simulink model "ctrl_ez"  (R2024b)
settings: configuration reference "CONFI" (kept outside this file)
InitFcn:
  | fidelity_pfc_vals;
  | wl=2*pi*50*150e-6;
  | 
  | gain_vac=1/(220*sqrt(2));
  | kpd = 5;
  | kpq = 5;
  | 
  | 
  | kid   =  1e2;
  | kiq   =  1e2;
  | 
  | kpvdc = .3;
  | kivdc =  .001;
values from neighbouring files (symbols this model uses):
  cos_th = cos(2*pi*50*t)    [fidelity_pfc_vals.m]
  sin_th = sin(2*pi*50*t)    [fidelity_pfc_vals.m]
  sin_th_vb = sin((2*pi*50*t)-(2*pi/3))    [fidelity_pfc_vals.m]
  sin_th_vc = sin((2*pi*50*t)+(2*pi/3))    [fidelity_pfc_vals.m]
  ts = 0.0001    [dic_pfc3ph.sldd]    (also in dictionary.sldd)
  tsw = 1/(fsw*1e3)    (= 1.53846153846e-05)    [fidelity_pfc_vals.m]
undefined symbols (not defined in the file or in its folder): DiscIntNeverNeededParam
libraries: mcbcontrolslib x18, simulink x5, dspswit3 x4, simulink_extras x2, slpidlib x2
(part 1 of 2)
settings Model: DataDictionary=dic_pfc3ph.sldd  Creator=Angel  LastModifiedBy=Angel
settings ConfigSetRef: SourceName=CONFI

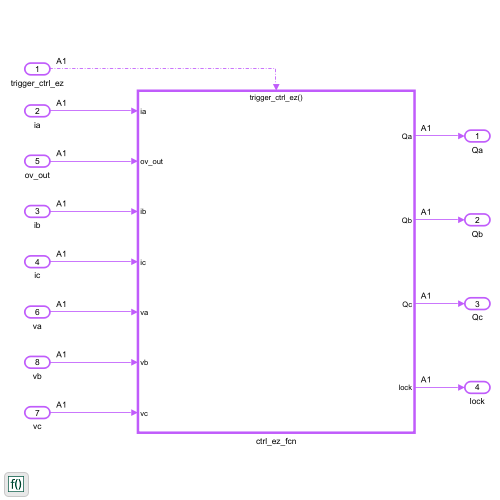
[thumbnail: Simulink's stored preview of the top-level diagram]
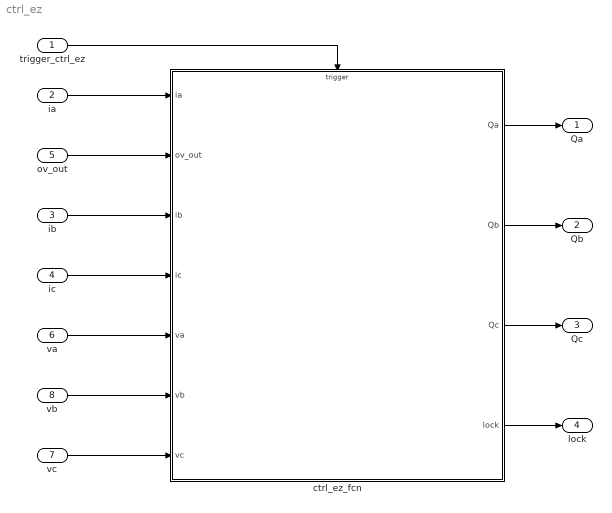
== system ctrl_ez ==
  trigger_ctrl_ez : Inport  OutputFunctionCall=on
  ia : Inport  Port=2
  ib : Inport  Port=3
  ic : Inport  Port=4
  ov_out : Inport  Port=5
  va : Inport  Port=6
  vc : Inport  Port=7
  vb : Inport  Port=8
  ctrl_ez_fcn : Subsystem
      settings: RTWSystemCode=Inline  RTWFcnNameOpts=Use subsystem name  RTWFileNameOpts=Use subsystem name  RTWMemSecFuncInitTerm=Default  RTWMemSecFuncExecute=Default
  Qa : Outport  PortDimensions=1
  Qb : Outport  Port=2
  Qc : Outport  Port=3
  lock : Outport  Port=4
  wires:
  ov_out/1 -> ctrl_ez_fcn/2(ov_out)
  trigger_ctrl_ez/1 -> ctrl_ez_fcn/Trigger
  va/1 -> ctrl_ez_fcn/5(va)
  ia/1 -> ctrl_ez_fcn/1(ia)
  vc/1 -> ctrl_ez_fcn/7(vc)
  ib/1 -> ctrl_ez_fcn/3(ib)
  vb/1 -> ctrl_ez_fcn/6(vb)
  ic/1 -> ctrl_ez_fcn/4(ic)
  ctrl_ez_fcn/1(Qa) -> Qa/1
  ctrl_ez_fcn/2(Qb) -> Qb/1
  ctrl_ez_fcn/3(Qc) -> Qc/1
  ctrl_ez_fcn/4(lock) -> lock/1

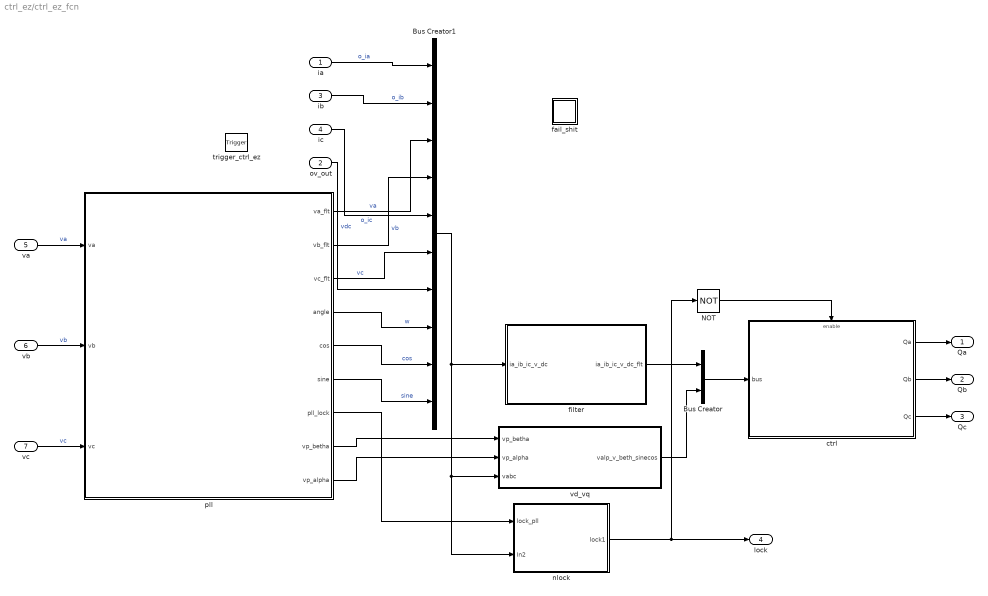
== system ctrl_ez/ctrl_ez_fcn ==
  ia : Inport  OutDataTypeStr=single
  ov_out : Inport  Port=2
  ib : Inport  Port=3  OutDataTypeStr=single
  ic : Inport  Port=4
  va : Inport  Port=5
  vb : Inport  Port=6
  vc : Inport  Port=7
  trigger_ctrl_ez : TriggerPort  TriggerType=function-call  VariantControl=(inherit)  PortDimensions=1
  Bus Creator : BusCreator  Inputs=2
  Bus Creator1 : BusCreator  Inputs=10
  NOT : Logic  Operator=NOT  IconShape=distinctive  AllPortsSameDT=off  OutDataTypeStr=boolean
  ctrl : Subsystem  TreatAsAtomicUnit=on
  fail_shit : Subsystem
  filter : Subsystem
  nlock : Subsystem
  pll : Subsystem
      settings: RTWSystemCode=Inline  RTWFcnNameOpts=Use subsystem name  RTWFileNameOpts=Use subsystem name  RTWMemSecFuncInitTerm=Default  RTWMemSecFuncExecute=Default
  vd_vq : Subsystem
  Qa : Outport
  Qb : Outport  Port=2
  Qc : Outport  Port=3
  lock : Outport  Port=4
  wires:
  ia/1 -> Bus Creator1/1  "o_ia"
  pll/3(vc_flt) -> Bus Creator1/6  "vc"
  pll/1(va_flt) -> Bus Creator1/3  "va"
  va/1 -> pll/1(va)  "va"
  ov_out/1 -> Bus Creator1/7  "vdc"
  vb/1 -> pll/2(vb)  "vb"
  ib/1 -> Bus Creator1/2  "o_ib"
  vc/1 -> pll/3(vc)  "vc"
  ic/1 -> Bus Creator1/5  "o_ic"
  ctrl/2(Qb) -> Qb/1
  pll/5(cos) -> Bus Creator1/9  "cos"
  pll/2(vb_flt) -> Bus Creator1/4  "vb"
  pll/6(sine) -> Bus Creator1/10  "sine"
  pll/4(angle) -> Bus Creator1/8  "w"
  pll/7(pll_lock) -> nlock/1(lock_pll)
  Bus Creator1/1 -> nlock/2(In2), vd_vq/3(vabc), filter/1(ia_ib_ic_v_dc)
  nlock/1(lock1) -> NOT/1, lock/1
  filter/1(ia_ib_ic_v_dc_flt) -> Bus Creator/1
  vd_vq/1(valp_v_beth_sinecos) -> Bus Creator/2
  NOT/1 -> ctrl/Enable
  Bus Creator/1 -> ctrl/1(bus)
  ctrl/1(Qa) -> Qa/1
  ctrl/3(Qc) -> Qc/1
  pll/8(vp_betha) -> vd_vq/1(vp_betha)
  pll/9(vp_alpha) -> vd_vq/2(vp_alpha)

== system ctrl_ez/ctrl_ez_fcn/ctrl ==
  bus : Inport
  Enable : EnablePort
  id_iq : Subsystem
  pi_ctrl : Subsystem
  svm : Subsystem
  Qa : Outport
  Qb : Outport  Port=2
  Qc : Outport  Port=3
  wires:
  id_iq/1(id) -> pi_ctrl/1(id)
  bus/1 -> svm/3(bus), pi_ctrl/3(bus), id_iq/1(In3)
  id_iq/2(iq) -> pi_ctrl/2(iq)
  svm/1(Qa) -> Qa/1
  svm/2(Qb) -> Qb/1
  svm/3(Qc) -> Qc/1
  pi_ctrl/1(d) -> svm/1(d)
  pi_ctrl/2(q) -> svm/2(q)

== system ctrl_ez/ctrl_ez_fcn/fail_shit ==
  pi+svpwm : Subsystem  Commented=on
  pi+svpwm1 : Subsystem  Commented=on

== system ctrl_ez/ctrl_ez_fcn/filter ==
  ia_ib_ic_v_dc : Inport
  Bus Creator : BusCreator  Inputs=3
  Bus Selector : BusSelector  OutputSignals=o_ia,o_ib,o_ic  OutputAsBus=on
  Data Store Memory : DataStoreMemory  DataStoreName=filter_IA  WriteAfterWriteMsg=warning  ShowAdditionalParam=off  StateMustResolveToSignalObject=on
  Data Store Memory1 : DataStoreMemory  DataStoreName=filter_IB  WriteAfterWriteMsg=warning  ShowAdditionalParam=off  StateMustResolveToSignalObject=on
  Data Store Memory2 : DataStoreMemory  DataStoreName=filter_IC  WriteAfterWriteMsg=warning  ShowAdditionalParam=off  StateMustResolveToSignalObject=on
  Data Store Write : DataStoreWrite  DataStoreName=filter_IA  IndexOptions=Index vector (dialog)  Indices=1  OutputSizes=1
  Data Store Write1 : DataStoreWrite  DataStoreName=filter_IB  IndexOptions=Index vector (dialog)  Indices=1  OutputSizes=1
  Data Store Write2 : DataStoreWrite  DataStoreName=filter_IC  IndexOptions=Index vector (dialog)  Indices=1  OutputSizes=1
  Demux : Demux  Outputs=3
  IIR Filter : mcbcontrolslib/IIR Filter  Commented=through  VariantControl=Low Pass Filter  VariantSelect=Low-pass  FilterConstantInputType=Specify via dialog  Filter_constant=.1  advancedSettings=on  Ts=1/8e3  cutOff_freq=141.4711
  ia_ib_ic_v_dc_flt : Outport
  wires:
  ia_ib_ic_v_dc/1 -> Bus Selector/1
  IIR Filter/1 -> Demux/1
  Bus Selector/1 -> IIR Filter/1
  Demux/1 -> Data Store Write/1, Bus Creator/1  "flt_ia"
  Demux/2 -> Data Store Write1/1, Bus Creator/2  "flt_ib"
  Demux/3 -> Data Store Write2/1, Bus Creator/3  "flt_ic"
  Bus Creator/1 -> ia_ib_ic_v_dc_flt/1

== system ctrl_ez/ctrl_ez_fcn/nlock ==
  lock_pll : Inport
  In2 : Inport  Port=2
  AND : Logic  IconShape=distinctive  AllPortsSameDT=off  OutDataTypeStr=boolean
  Bus Selector : BusSelector  OutputSignals=w
  Constant : Constant  Value=0  OutDataTypeStr=boolean  SampleTime=-1
  Equal : RelationalOperator  Operator=>  OutDataTypeStr=boolean  RndMeth=Simplest  InputSameDT=off
  Memory : Memory  InitialCondition=1  InheritSampleTime=on
  Pi1 : Constant  Value=0  OutDataTypeStr=single  SampleTime=-1
  Switch : Switch  Criteria=u2 > Threshold  SaturateOnIntegerOverflow=off  InputSameDT=off
  lock1 : Outport
  wires:
  Switch/1 -> lock1/1, Memory/1
  Constant/1 -> Switch/1
  Memory/1 -> Switch/3
  In2/1 -> Bus Selector/1
  Bus Selector/1 -> Equal/1  "<w>"
  Equal/1 -> AND/1
  Pi1/1 -> Equal/2
  lock_pll/1 -> AND/2
  AND/1 -> Switch/2

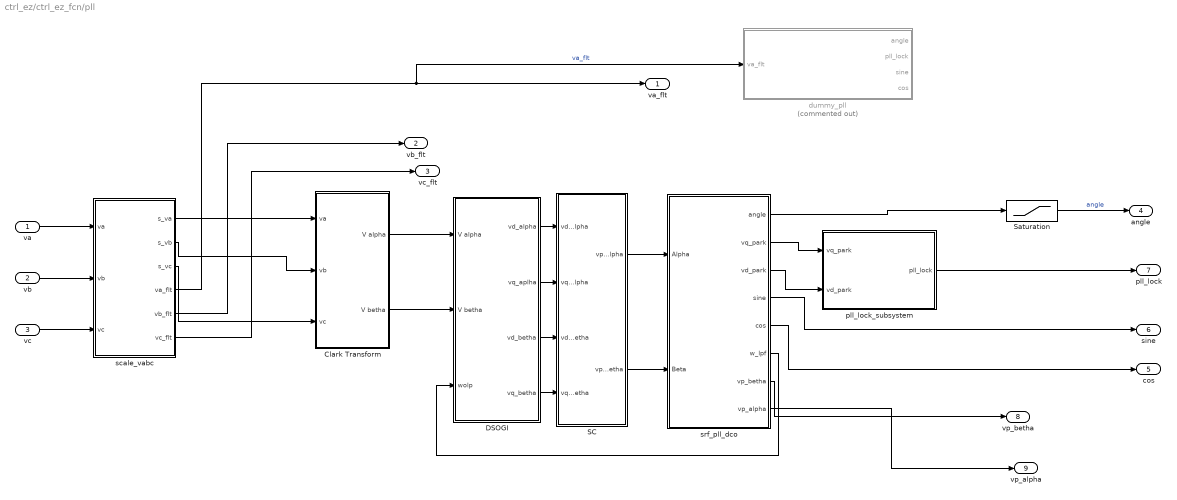
== system ctrl_ez/ctrl_ez_fcn/pll ==
  va : Inport  OutDataTypeStr=single
  vb : Inport  Port=2  OutDataTypeStr=single
  vc : Inport  Port=3  OutDataTypeStr=single
  Clark Transform : Subsystem  SystemSampleTime=ts
  DSOGI : Subsystem  SystemSampleTime=ts
  SC : Subsystem  SystemSampleTime=ts
  Saturation : Saturate  UpperLimit=2*pi  LowerLimit=0
  dummy_pll : Subsystem  Commented=on
  pll_lock_subsystem : Subsystem
  scale_vabc : Subsystem
  srf_pll_dco : Subsystem
  va_flt : Outport
  vb_flt : Outport  Port=2
  vc_flt : Outport  Port=3
  angle : Outport  Port=4
  cos : Outport  Port=5
  sine : Outport  Port=6
  pll_lock : Outport  Port=7
  vp_betha : Outport  Port=8
  vp_alpha : Outport  Port=9
  wires:
  vb/1 -> scale_vabc/2(vb)
  scale_vabc/3(s_vc) -> Clark Transform/3(vc)
  scale_vabc/2(s_vb) -> Clark Transform/2(vb)
  srf_pll_dco/5(cos) -> cos/1
  pll_lock_subsystem/1(pll_lock) -> pll_lock/1
  srf_pll_dco/2(vq_park) -> pll_lock_subsystem/1(vq_park)
  SC/2(vp_betha) -> srf_pll_dco/2(Beta)
  SC/1(vp_alpha) -> srf_pll_dco/1(Alpha)
  DSOGI/2(vq_aplha) -> SC/2(vq_sogi_alpha)
  DSOGI/1(vd_alpha) -> SC/1(vd_sogi_alpha)
  srf_pll_dco/3(vd_park) -> pll_lock_subsystem/2(vd_park)
  srf_pll_dco/6(w_lpf) -> DSOGI/3(wolp)
  va/1 -> scale_vabc/1(va)
  Clark Transform/2(V betha) -> DSOGI/2(V betha)
  scale_vabc/1(s_va) -> Clark Transform/1(va)
  srf_pll_dco/4(sine) -> sine/1
  srf_pll_dco/1(angle) -> Saturation/1
  DSOGI/3(vd_betha) -> SC/3(vd_sogi_betha)
  Clark Transform/1(V alpha) -> DSOGI/1(V alpha)
  DSOGI/4(vq_betha) -> SC/4(vq_sogi_betha)
  vc/1 -> scale_vabc/3(vc)
  scale_vabc/4(va_flt) -> dummy_pll/1(va_flt), va_flt/1  "va_flt"
  scale_vabc/5(vb_flt) -> vb_flt/1
  scale_vabc/6(vc_flt) -> vc_flt/1
  Saturation/1 -> angle/1  "angle"
  srf_pll_dco/7(vp_betha) -> vp_betha/1
  srf_pll_dco/8(vp_alpha) -> vp_alpha/1

== system ctrl_ez/ctrl_ez_fcn/vd_vq ==
  vp_betha : Inport
  vp_alpha : Inport  Port=2
  vabc : Inport  Port=3
  Bus Creator : BusCreator  Inputs=3
  Bus Creator1 : BusCreator  Inputs=2
  Bus Selector : BusSelector  OutputSignals=w,vc,vb,va,cos,sine
  Clarke Transform : mcbcontrolslib/Clarke Transform  Commented=on  VariantControl=Variant2  PhaseInput=Three inputs  EnPowerInv=on
      settings: LibrarySourceBlock=mcbhdllib/Controls/Math Transforms/Clarke Transform
  Demux : Demux  Commented=on  Outputs=3
  Mux : Mux  Commented=on  Inputs=3
  Park Transform : mcbcontrolslib/Park Transform  Commented=on  PhaseInput=Two inputs  AxisAlignment=Q-axis  ThetaInput=Sine and Cosine electrical position  AngleInput=Radians  N_points=1024
  Terminator : Terminator  Commented=on
  park_tf : MATLAB Function  Commented=on  TreatAsAtomicUnit=on  VariantControl=false()
  valp_v_beth_sinecos : Outport
  wires:
  vabc/1 -> Bus Creator1/2, Bus Selector/1
  vp_alpha/1 -> Bus Creator/1  "vd_"
  vp_betha/1 -> Bus Creator/2  "vq_"
  Bus Selector/1 -> Bus Creator/3  "<w>"
  Bus Creator/1 -> Bus Creator1/1
  Bus Creator1/1 -> valp_v_beth_sinecos/1
  Bus Selector/5 -> Park Transform/4, park_tf/4(cos_th_k_1)  "<cos>"
  Bus Selector/6 -> Park Transform/3, park_tf/3(sin_th_k_1)  "<sine>"
  Mux/1 -> Clarke Transform/1
  Demux/3 -> Terminator/1
  Clarke Transform/1 -> Demux/1
  Demux/1 -> park_tf/1(vp_alpha)
  Demux/2 -> park_tf/2(vp_betha)
  Bus Selector/2 -> Mux/3  "<vc>"
  Bus Selector/3 -> Mux/2  "<vb>"
  Bus Selector/4 -> Mux/1  "<va>"

== system ctrl_ez/ctrl_ez_fcn/ctrl/id_iq ==
  In3 : Inport
  Bus Selector1 : BusSelector  OutputSignals=signal1.flt_ia,signal1.flt_ib,signal1.flt_ic,signal2.signal2.cos,signal2.signal2.sine
  Clarke Transform : mcbcontrolslib/Clarke Transform  VariantControl=Variant2  PhaseInput=Three inputs  EnPowerInv=on
      settings: LibrarySourceBlock=mcbhdllib/Controls/Math Transforms/Clarke Transform
  Demux1 : Demux  Outputs=3
  Mux : Mux  Inputs=3
  Terminator1 : Terminator
  park_tf : MATLAB Function  TreatAsAtomicUnit=on  VariantControl=false()
  id : Outport
  iq : Outport  Port=2
  wires:
  In3/1 -> Bus Selector1/1
  Demux1/2 -> park_tf/2(vp_betha)  "iq"
  Clarke Transform/1 -> Demux1/1
  Bus Selector1/1 -> Mux/1  "<flt_ia>"
  Mux/1 -> Clarke Transform/1
  Bus Selector1/2 -> Mux/2  "<flt_ib>"
  Bus Selector1/3 -> Mux/3  "<flt_ic>"
  Demux1/1 -> park_tf/1(vp_alpha)  "id"
  Demux1/3 -> Terminator1/1
  park_tf/1(vd_park) -> id/1  "id"
  park_tf/2(vq_park) -> iq/1  "iq"
  Bus Selector1/4 -> park_tf/4(cos_th_k_1)  "<cos>"
  Bus Selector1/5 -> park_tf/3(sin_th_k_1)  "<sine>"

== system ctrl_ez/ctrl_ez_fcn/ctrl/pi_ctrl ==
  id : Inport
  iq : Inport  Port=2
  bus : Inport  Port=3
  Bus Selector2 : BusSelector  OutputSignals=signal2.signal1.vd_,signal2.signal1.vq_,signal2.signal2.vdc
  Constant : Constant  Value=650  OutDataTypeStr=single  SampleTime=-1
  Constant1 : Constant  Value=0  OutDataTypeStr=single  SampleTime=-1
  Gain : Gain  Gain=wl
  Gain1 : Gain  Gain=wl
  Sum1 : Sum  Inputs=|+-
  Sum2 : Sum  Inputs=|+-
  Sum3 : Sum  Inputs=++-
  Sum4 : Sum  Inputs=-|+||
  Sum5 : Sum  Inputs=+--
  id_ctrl : Subsystem  SystemSampleTime=tsw
  iq_ctrl : Subsystem  SystemSampleTime=tsw
  speed_ctrl : Subsystem  SystemSampleTime=tsw
  d : Outport
  q : Outport  Port=2
  wires:
  Constant/1 -> Sum1/1
  Sum1/1 -> speed_ctrl/1(i_error)  "vdc_error"
  iq/1 -> Sum4/1, Gain/1  "iq"
  speed_ctrl/1(I_D_CTRL_VDC) -> Sum2/1  "id_ctrl"
  Constant1/1 -> Sum4/2  "vq_ctrl"
  id/1 -> Sum2/2, Gain1/1  "id"
  Sum4/1 -> iq_ctrl/1(i_error)  "iq_error"
  Sum2/1 -> id_ctrl/1(i_error)  "id_error"
  Gain1/1 -> Sum5/2  "idwl"
  iq_ctrl/1(v_ind) -> Sum5/3  "vq_ctrl"
  Gain/1 -> Sum3/2  "iqwl"
  id_ctrl/1(v_ind) -> Sum3/3  "vd_ctrl"
  Sum5/1 -> q/1  "vq_ctrl"
  Sum3/1 -> d/1  "vd_ctrl"
  bus/1 -> Bus Selector2/1
  Bus Selector2/3 -> Sum1/2  "<vdc>"
  Bus Selector2/1 -> Sum3/1  "<vd_>"
  Bus Selector2/2 -> Sum5/1  "<vq_>"

== system ctrl_ez/ctrl_ez_fcn/ctrl/svm ==
  d : Inport
  q : Inport  Port=2
  bus : Inport  Port=3
  Bus Selector : BusSelector  OutputSignals=signal2.signal2.cos,signal2.signal2.sine,signal2.signal2.w,signal2.signal2.vdc
  mine_invpark_tf : MATLAB Function  TreatAsAtomicUnit=on  VariantControl=false()
  pi+svpwm1 : Subsystem  Commented=on
  relat_time : Subsystem
  section_cal : Subsystem
  threshold : Subsystem
  Qa : Outport
  Qb : Outport  Port=2
  Qc : Outport  Port=3
  wires:
  mine_invpark_tf/1(vp_alpha) -> section_cal/2(v_alp)  "vind_alp"
  mine_invpark_tf/2(vp_betha) -> section_cal/3(v_bet)  "vind_bet"
  section_cal/1(alpha) -> relat_time/2(alpha)
  threshold/3(qc) -> Qc/1
  section_cal/2(oddsect) -> relat_time/3(odd_section)
  threshold/2(qb) -> Qb/1
  section_cal/3(vs_mag) -> relat_time/4(vs_mag)
  relat_time/1(ta_tb_t0) -> threshold/1(ta_tb_t0)
  section_cal/4(SA SB SC) -> threshold/2(SA SB SC)
  threshold/1(qa) -> Qa/1
  bus/1 -> Bus Selector/1
  d/1 -> mine_invpark_tf/1(vd_park)
  q/1 -> mine_invpark_tf/2(vq_park)
  Bus Selector/1 -> mine_invpark_tf/4(cos_th_k_1)  "<cos>"
  Bus Selector/2 -> mine_invpark_tf/3(sin_th_k_1)  "<sine>"
  Bus Selector/3 -> section_cal/1(<w>)  "<w>"
  Bus Selector/4 -> relat_time/1(vdc)  "<vdc>"

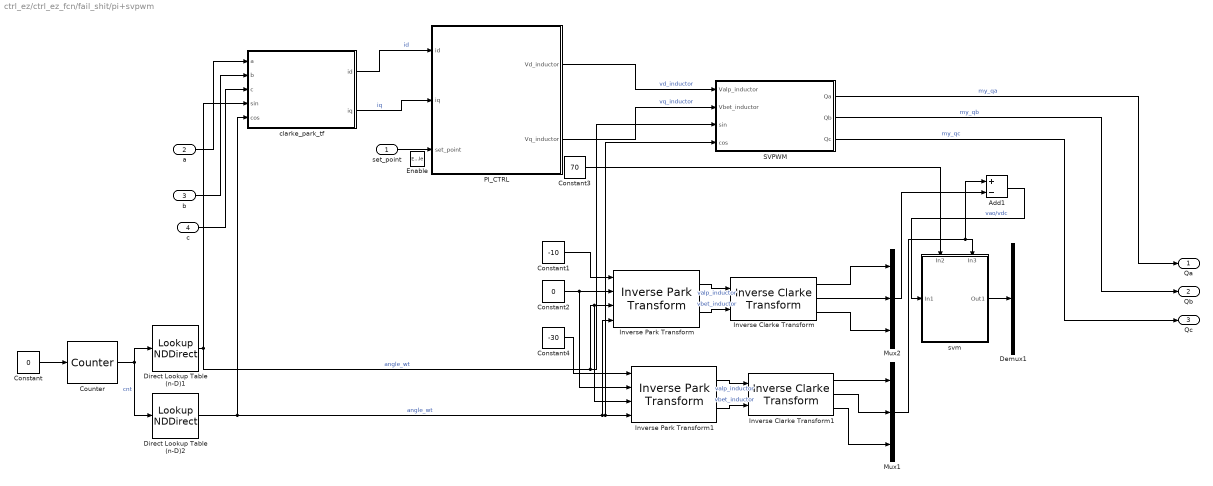
== system ctrl_ez/ctrl_ez_fcn/fail_shit/pi+svpwm ==
  set_point : Inport
  a : Inport  Port=2
  b : Inport  Port=3
  c : Inport  Port=4
  Enable : EnablePort
  Add1 : Sum  Inputs=+-
  Constant : Constant  Value=0  SampleTime=-1
  Constant1 : Constant  Value=-10
  Constant2 : Constant  Value=0
  Constant3 : Constant  Value=70
  Constant4 : Constant  Value=-30
  Counter : dspswit3/Counter  Direction=Up  CountEvent=Free running  CounterSize=User defined  MaxCount=(.01/tsw)+1  InitialCount=0  Output=Count  HitValue=32  ResetInput=on  SamplesPerFrame=1  Ts=-1  CntDtype=uint32  HitDtype=Logical
  Demux1 : Demux  Outputs=3
  Direct Lookup Table (n-D)1 : LookupNDDirect  NumberOfTableDimensions=1  Table=single(sin_th);  RemoveProtectionInput=on  TableDataTypeStr=single
  Direct Lookup Table (n-D)2 : LookupNDDirect  NumberOfTableDimensions=1  Table=single(cos_th);  RemoveProtectionInput=on  TableDataTypeStr=single
  Inverse Clarke Transform : mcbcontrolslib/Inverse Clarke Transform  PhaseInput=Two inputs  EnPowerInv=off
      settings: LibrarySourceBlock=mcbhdllib/Controls/Math Transforms/Inverse Clarke Transform
  Inverse Clarke Transform1 : mcbcontrolslib/Inverse Clarke Transform  PhaseInput=Two inputs  EnPowerInv=off
      settings: LibrarySourceBlock=mcbhdllib/Controls/Math Transforms/Inverse Clarke Transform
  Inverse Park Transform : mcbcontrolslib/Inverse Park Transform  PhaseInput=Two inputs  AxisAlignment=D-axis  ThetaInput=Sine and Cosine electrical position  AngleInput=Per-unit  N_points=1024
      settings: LibrarySourceBlock=mcbhdllib/Controls/Math Transforms/Inverse Park Transform
  Inverse Park Transform1 : mcbcontrolslib/Inverse Park Transform  PhaseInput=Two inputs  AxisAlignment=D-axis  ThetaInput=Sine and Cosine electrical position  AngleInput=Per-unit  N_points=1024
      settings: LibrarySourceBlock=mcbhdllib/Controls/Math Transforms/Inverse Park Transform
  Mux1 : Mux  Inputs=3
  Mux2 : Mux  Inputs=3
  PI_CTRL : Subsystem  SystemSampleTime=tsw
  SVPWM : Subsystem  SystemSampleTime=tsw
  clarke_park_tf : Subsystem
  svm : Subsystem
      settings: PortSchema="{\"entries\":[{\"content\":{\"sides\":[{\"content\":{\"connectorIds\":[\"In1\"]},\"type\":\"ConnectorPlacement.EquallySpacedRectSide\",\"uuid\":\"3e008ee5-59f8-4da6-a2e7-d375939bf865\"},{\"content\":{\"connectorIds\":[\"Out1\"],\"side\":\"RIGHT\"},\"type\":\"ConnectorPlacement.EquallySpacedRectSide\",\"uuid\":\"8b37db03-1d3b-40e7-b6c7-a20c319c3381\"},{\"content\":{\"connectorIds\":[\"In2\",\"In3\"],\"side\":\"TOP\"},\"type\":\"ConnectorPlacement.EquallySpacedRectSide\",\"uuid\":\"db383d90-c1d4-4862-ad96-70764e497fba\"}]},\"type\":\"ConnectorPlacement.EquallySpacedConnector\",\"uuid\":\"69b3b40e-ea56-4f3d-9cab-f35d699fcec1\"}],\"packageUris\":[\"http://schema.mathworks.com/mf0/Connector/R2020b\"],\"version\":\"1.0\"}"
  Qa : Outport
  Qb : Outport  Port=2
  Qc : Outport  Port=3
  wires:
  b/1 -> clarke_park_tf/2(b)
  c/1 -> clarke_park_tf/3(c)
  Constant/1 -> Counter/1
  Counter/1 -> Direct Lookup Table (n-D)2/1, Direct Lookup Table (n-D)1/1  "cnt"
  set_point/1 -> PI_CTRL/3(set_point)
  a/1 -> clarke_park_tf/1(a)
  clarke_park_tf/1(id) -> PI_CTRL/1(id)  "id"
  Direct Lookup Table (n-D)2/1 -> clarke_park_tf/5(cos), SVPWM/4(cos), Inverse Park Transform1/4, Inverse Park Transform/4  "angle_wt"
  Direct Lookup Table (n-D)1/1 -> SVPWM/3(sin), Inverse Park Transform1/3, Inverse Park Transform/3, clarke_park_tf/4(sin)  "angle_wt"
  clarke_park_tf/2(iq) -> PI_CTRL/2(iq)  "iq"
  Constant1/1 -> Inverse Park Transform/1
  Constant2/1 -> Inverse Park Transform1/2, Inverse Park Transform/2
  Constant3/1 -> svm/2(In2)
  Add1/1 -> svm/1(In1)  "vao/vdc"
  Mux2/1 -> Add1/2
  svm/1(Out1) -> Demux1/1
  Inverse Park Transform/2 -> Inverse Clarke Transform/2  "vbet_inductor"
  Inverse Park Transform/1 -> Inverse Clarke Transform/1  "valp_inductor"
  Inverse Clarke Transform/2 -> Mux2/2
  Inverse Clarke Transform/3 -> Mux2/3
  Inverse Clarke Transform/1 -> Mux2/1
  Inverse Park Transform1/1 -> Inverse Clarke Transform1/1  "valp_inductor"
  Inverse Park Transform1/2 -> Inverse Clarke Transform1/2  "vbet_inductor"
  Inverse Clarke Transform1/1 -> Mux1/1
  Inverse Clarke Transform1/2 -> Mux1/2
  Inverse Clarke Transform1/3 -> Mux1/3
  Mux1/1 -> Add1/1, svm/3(In3)
  Constant4/1 -> Inverse Park Transform1/1
  PI_CTRL/1(Vd_inductor) -> SVPWM/1(Valp_inductor)  "vd_inductor"
  PI_CTRL/2(Vq_inductor) -> SVPWM/2(Vbet_inductor)  "vq_inductor"
  SVPWM/1(Qa) -> Qa/1  "my_qa"
  SVPWM/2(Qb) -> Qb/1  "my_qb"
  SVPWM/3(Qc) -> Qc/1  "my_qc"

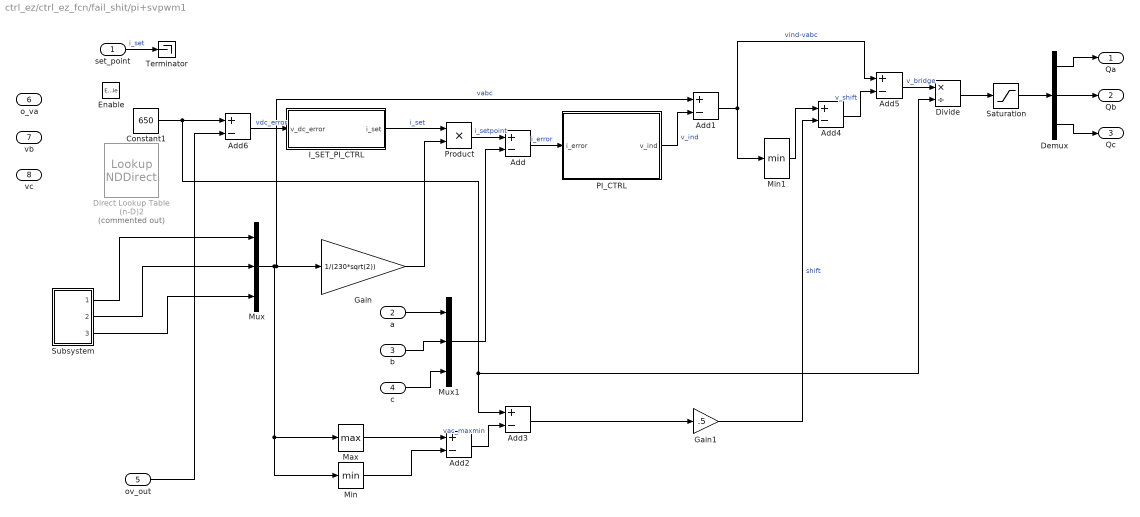
== system ctrl_ez/ctrl_ez_fcn/fail_shit/pi+svpwm1 ==
  set_point : Inport
  a : Inport  Port=2
  b : Inport  Port=3
  c : Inport  Port=4
  ov_out : Inport  Port=5
  o_va : Inport  Port=6
  vb : Inport  Port=7
  vc : Inport  Port=8
  Enable : EnablePort
  Add{,1..6} (7 alike) : Sum  Inputs=+-
  Constant1 : Constant  Value=650  VectorParams1D=off  OutDataTypeStr=single  SampleTime=-1
  Demux : Demux  Outputs=3
  Direct Lookup Table (n-D)2 : LookupNDDirect  Commented=on  NumberOfTableDimensions=1  Table=single(cos_th);  RemoveProtectionInput=on  TableDataTypeStr=single
  Divide : Product  Inputs=*/
  Gain : Gain  Gain=1/(230*sqrt(2))
  Gain1 : Gain  Gain=.5
  I_SET_PI_CTRL : Subsystem  SystemSampleTime=tsw
  Max : MinMax  Function=max
  Min : MinMax
  Min1 : MinMax
  Mux : Mux  Inputs=3
  Mux1 : Mux  Inputs=3
  PI_CTRL : Subsystem  SystemSampleTime=tsw
  Product : Product
  Saturation : Saturate  UpperLimit=.97  LowerLimit=.03
  Subsystem : Subsystem
  Terminator : Terminator
  Qa : Outport
  Qb : Outport  Port=2
  Qc : Outport  Port=3
  wires:
  Constant1/1 -> Add3/1, Divide/2, Add6/1
  ov_out/1 -> Add6/2
  Gain/1 -> Product/2
  Add6/1 -> I_SET_PI_CTRL/1(v_dc_error)  "vdc_error"
  b/1 -> Mux1/2
  Mux/1 -> Max/1, Min/1, Add1/1, Gain/1  "vabc"
  set_point/1 -> Terminator/1  "i_set"
  a/1 -> Mux1/1
  c/1 -> Mux1/3
  Max/1 -> Add2/1
  Min/1 -> Add2/2
  Product/1 -> Add/1  "i_setpoint"
  Mux1/1 -> Add/2
  Add2/1 -> Add3/2  "vac_maxmin"
  Add/1 -> PI_CTRL/1(i_error)  "i_error"
  Add3/1 -> Gain1/1
  PI_CTRL/1(v_ind) -> Add1/2  "v_ind"
  Add1/1 -> Add5/1, Min1/1  "vind-vabc"
  Gain1/1 -> Add4/2  "shift"
  Min1/1 -> Add4/1
  Add4/1 -> Add5/2  "v_shift"
  Add5/1 -> Divide/1  "v_bridge"
  Divide/1 -> Saturation/1
  Demux/2 -> Qb/1
  Demux/1 -> Qa/1
  Saturation/1 -> Demux/1
  Demux/3 -> Qc/1
  I_SET_PI_CTRL/1(i_set) -> Product/1  "i_set"
  Subsystem/1(angle_wt) -> Mux/1
  Subsystem/2(angle_wt1) -> Mux/2
  Subsystem/3(angle_wt2) -> Mux/3

== system ctrl_ez/ctrl_ez_fcn/pll/Clark Transform ==
  va : Inport  OutDataTypeStr=single
  vb : Inport  Port=2  OutDataTypeStr=single
  vc : Inport  Port=3  OutDataTypeStr=single
  Clarke Transform : mcbcontrolslib/Clarke Transform  VariantControl=Variant2  PhaseInput=Three inputs  EnPowerInv=on
      settings: LibrarySourceBlock=mcbhdllib/Controls/Math Transforms/Clarke Transform
  Demux : Demux  Outputs=3
  Mux : Mux  Inputs=3
  Terminator : Terminator
  V alpha : Outport
  V betha : Outport  Port=2
  wires:
  vb/1 -> Mux/2
  va/1 -> Mux/1
  Demux/3 -> Terminator/1
  Demux/2 -> V betha/1  "V betha_pll"
  Demux/1 -> V alpha/1  "V alpha_pll"
  vc/1 -> Mux/3
  Mux/1 -> Clarke Transform/1
  Clarke Transform/1 -> Demux/1

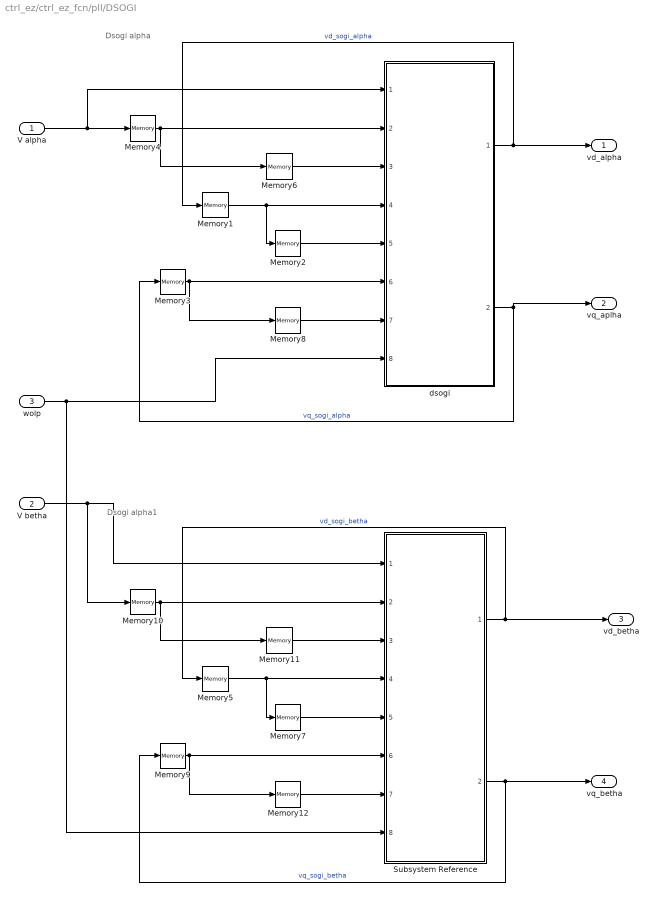
== system ctrl_ez/ctrl_ez_fcn/pll/DSOGI ==
  note: Dsogi alpha1
  note: Dsogi alpha
  V alpha : Inport  OutDataTypeStr=single
  V betha : Inport  Port=2  OutDataTypeStr=single
  wolp : Inport  Port=3  OutDataTypeStr=single
  Memory{1..12} (12 alike) : Memory  InheritSampleTime=on
  Subsystem Reference : Subsystem  ReferencedSubsystem=dsogi
  dsogi : Subsystem  ReferencedSubsystem=dsogi
  vd_alpha : Outport
  vq_aplha : Outport  Port=2
  vd_betha : Outport  Port=3
  vq_betha : Outport  Port=4
  wires:
  dsogi/2 -> vq_aplha/1, Memory3/1  "vq_sogi_alpha"
  dsogi/1 -> vd_alpha/1, Memory1/1  "vd_sogi_alpha"
  Memory8/1 -> dsogi/7
  Memory2/1 -> dsogi/5
  Memory6/1 -> dsogi/3
  Memory3/1 -> dsogi/6, Memory8/1
  Memory1/1 -> dsogi/4, Memory2/1
  Memory4/1 -> dsogi/2, Memory6/1
  V alpha/1 -> dsogi/1, Memory4/1
  Subsystem Reference/2 -> vq_betha/1, Memory9/1  "vq_sogi_betha"
  Subsystem Reference/1 -> vd_betha/1, Memory5/1  "vd_sogi_betha"
  wolp/1 -> Subsystem Reference/8, dsogi/8
  Memory12/1 -> Subsystem Reference/7
  Memory7/1 -> Subsystem Reference/5
  Memory11/1 -> Subsystem Reference/3
  V betha/1 -> Subsystem Reference/1, Memory10/1
  Memory10/1 -> Subsystem Reference/2, Memory11/1
  Memory5/1 -> Subsystem Reference/4, Memory7/1
  Memory9/1 -> Subsystem Reference/6, Memory12/1

== system ctrl_ez/ctrl_ez_fcn/pll/SC ==
  note: c=0.5*(a+b);
  note: c=0.5*(a-b);
  note: NSC
  vd_sogi_alpha : Inport  OutDataTypeStr=single
  vq_sogi_alpha : Inport  Port=2  OutDataTypeStr=single
  vd_sogi_betha : Inport  Port=3  OutDataTypeStr=single
  vq_sogi_betha : Inport  Port=4  OutDataTypeStr=single
  Add : Sum  Inputs=+-
  Add1 : Sum
  Gain : Gain  Gain=.5  OutDataTypeStr=single
  Gain1 : Gain  Gain=.5  OutDataTypeStr=single
  Gain2 : Gain  Commented=on  Gain=-1
  Terminator : Terminator  Commented=on
  Terminator1 : Terminator  Commented=on
  Terminator2 : Terminator  Commented=on
  a-b : MATLAB Function  TreatAsAtomicUnit=on  VariantControl=false()
      settings: RTWSystemCode=Inline
  sum : MATLAB Function  TreatAsAtomicUnit=on  VariantControl=false()
  sum1 : MATLAB Function  TreatAsAtomicUnit=on  VariantControl=false()
  sum2 : MATLAB Function  TreatAsAtomicUnit=on  VariantControl=false()
      settings: RTWSystemCode=Inline
  vp_alpha : Outport
  vp_betha : Outport  Port=2
  wires:
  vd_sogi_betha/1 -> Add1/2, a-b/1(a)  "a"
  Gain1/1 -> vp_betha/1, sum1/1(a)  "vp_betha"
  vd_sogi_alpha/1 -> Add/1, Gain2/1, sum2/1(a)
  sum/1(c) -> Terminator1/1  "vz_alp"
  Add1/1 -> Gain1/1
  vq_sogi_alpha/1 -> Add1/1, a-b/2(b)
  Add/1 -> Gain/1
  Gain/1 -> sum/1(a), vp_alpha/1  "vp_alpha"
  vq_sogi_betha/1 -> Add/2, sum2/2(b)  "b"
  Gain2/1 -> Terminator2/1  "nvq_sogi_alpha"
  sum1/1(c) -> Terminator/1  "vz_bet"
  a-b/1(c) -> sum1/2(b)  "Vn_betha"
  sum2/1(c) -> sum/2(b)  "Vn_alpha"

== system ctrl_ez/ctrl_ez_fcn/pll/dummy_pll ==
  va_flt : Inport
  Constant : Constant  Value=0  OutDataTypeStr=boolean  SampleTime=-1
  Counter : dspswit3/Counter  Direction=Up  CountEvent=Free running  CounterSize=User defined  MaxCount=200  InitialCount=0  Output=Count  HitValue=32  ResetInput=on  SamplesPerFrame=1  Ts=-1  CntDtype=uint32  HitDtype=Logical
  Data Type Conversion : DataTypeConversion  OutDataTypeStr=single  SaturateOnIntegerOverflow=off  RndMeth=Floor
  Memory : Memory  InitialCondition=1  InheritSampleTime=on
  NOT : Logic  Operator=NOT  IconShape=distinctive  AllPortsSameDT=off  OutDataTypeStr=boolean
  Switch : Switch  Criteria=u2 > Threshold  SaturateOnIntegerOverflow=off  InputSameDT=off
  angle_lookup_table2 : LookupNDDirect  NumberOfTableDimensions=1  Table=single(2*pi*50*t)  RemoveProtectionInput=on
  cos_lookup_table1 : LookupNDDirect  NumberOfTableDimensions=1  Table=single(cos_th)  RemoveProtectionInput=on
  sine_lookup_table : LookupNDDirect  NumberOfTableDimensions=1  Table=single(sin_th)  RemoveProtectionInput=on
  zcd : Subsystem  SystemSampleTime=tsw
  angle : Outport
  pll_lock : Outport  Port=2
  sine : Outport  Port=3
  cos : Outport  Port=4
  wires:
  va_flt/1 -> zcd/1(v_ac)
  Memory/1 -> Switch/3
  Switch/1 -> NOT/1, Counter/1, Memory/1
  zcd/1(zcd) -> Switch/2
  Constant/1 -> Switch/1
  cos_lookup_table1/1 -> cos/1
  sine_lookup_table/1 -> sine/1
  NOT/1 -> Data Type Conversion/1
  Counter/1 -> angle_lookup_table2/1, cos_lookup_table1/1, sine_lookup_table/1
  angle_lookup_table2/1 -> angle/1
  Data Type Conversion/1 -> pll_lock/1  "pll_lock"

== system ctrl_ez/ctrl_ez_fcn/pll/pll_lock_subsystem ==
  vq_park : Inport
  vd_park : Inport  Port=2
  AND : Logic  IconShape=distinctive  AllPortsSameDT=off  OutDataTypeStr=boolean
  Constant2 : Constant  Value=.75  OutDataTypeStr=single  SampleTime=-1
  Constant3 : Constant  Value=1.4  OutDataTypeStr=single  SampleTime=-1
  Data Type Conversion : DataTypeConversion  OutDataTypeStr=single  SaturateOnIntegerOverflow=off  RndMeth=Floor
  Difference : simulink/Discrete/Difference  Commented=on  ICPrevInput=0.0  OutMin=[]  OutMax=[]  OutDataType=fixdt(1, 16)  OutScaling=2^-10  DoSatur=off
  Equal2 : RelationalOperator  OutDataTypeStr=boolean  RndMeth=Simplest  InputSameDT=off
  Equal3 : RelationalOperator  OutDataTypeStr=boolean  RndMeth=Simplest  InputSameDT=off
  MATLAB Function : MATLAB Function  TreatAsAtomicUnit=on
  Mux : Mux  Commented=on  Inputs=2
  cnt : Memory  InheritSampleTime=on
  pll_lock : Outport
  wires:
  Equal3/1 -> AND/2
  Constant2/1 -> Equal2/2
  Constant3/1 -> Equal3/1
  vd_park/1 -> Equal3/2, Equal2/1, Mux/2
  vq_park/1 -> Mux/1
  Equal2/1 -> AND/1
  Mux/1 -> Difference/1
  cnt/1 -> MATLAB Function/2(cnt_1)
  AND/1 -> MATLAB Function/1(u)  "pll_lock"
  MATLAB Function/2(cnt) -> cnt/1
  Data Type Conversion/1 -> pll_lock/1
  MATLAB Function/1(y) -> Data Type Conversion/1  "pll_lock"

== system ctrl_ez/ctrl_ez_fcn/pll/scale_vabc ==
  va : Inport
  vb : Inport  Port=2
  vc : Inport  Port=3
  Demux : Demux  Outputs=3
  Demux1 : Demux  Outputs=3
  Gain : Gain  Gain=gain_vac  OutDataTypeStr=single
  IIR Filter : mcbcontrolslib/IIR Filter  Commented=through  VariantControl=Low Pass Filter  VariantSelect=Low-pass  FilterConstantInputType=Specify via dialog  Filter_constant=.1  advancedSettings=on  Ts=1/8e3  cutOff_freq=141.4711
  Mux : Mux  Inputs=3
  s_va : Outport
  s_vb : Outport  Port=2
  s_vc : Outport  Port=3
  va_flt : Outport  Port=4
  vb_flt : Outport  Port=5
  vc_flt : Outport  Port=6
  wires:
  va/1 -> Mux/1
  Gain/1 -> Demux/1
  vb/1 -> Mux/2
  vc/1 -> Mux/3
  Mux/1 -> IIR Filter/1
  Demux/2 -> s_vb/1
  Demux/1 -> s_va/1
  Demux/3 -> s_vc/1
  IIR Filter/1 -> Demux1/1, Gain/1
  Demux1/1 -> va_flt/1
  Demux1/2 -> vb_flt/1
  Demux1/3 -> vc_flt/1

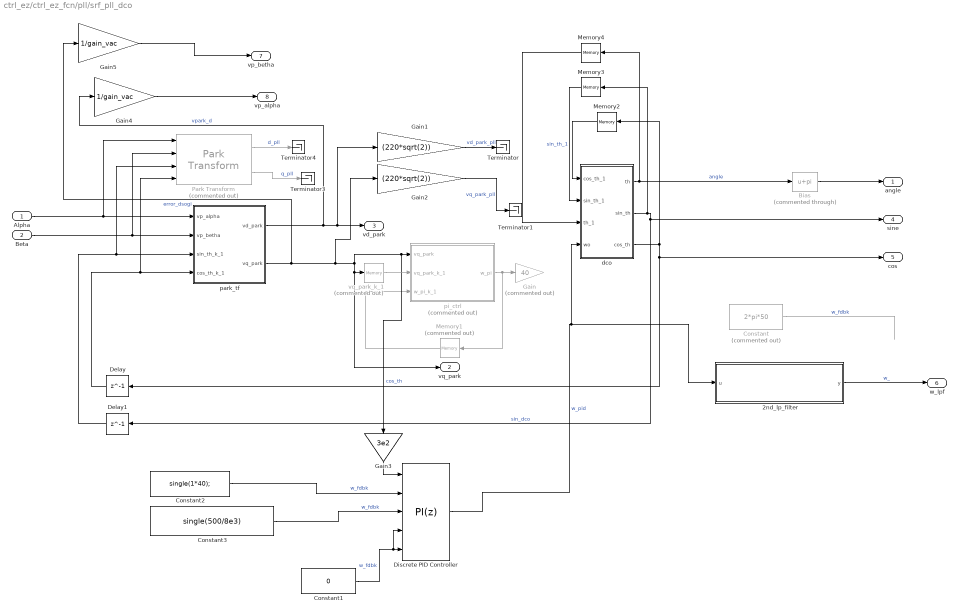
== system ctrl_ez/ctrl_ez_fcn/pll/srf_pll_dco ==
  Alpha : Inport  OutDataTypeStr=single
  Beta : Inport  Port=2  OutDataTypeStr=single
  2nd_lp_filter : Subsystem
  Bias : Bias  Commented=through  Bias=pi  SaturateOnIntegerOverflow=off
  Constant : Constant  Commented=on  Value=2*pi*50  OutDataTypeStr=single  SampleTime=-1
  Constant1 : Constant  Value=0  OutDataTypeStr=single  SampleTime=-1
  Constant2 : Constant  Value=single(1*40);  OutDataTypeStr=single  SampleTime=-1
  Constant3 : Constant  Value=single(500/8e3)  OutDataTypeStr=single  SampleTime=-1
  Delay : Delay  DelayLength=1
  Delay1 : Delay  DelayLength=1
  Discrete PID Controller : slpidlib/PID Controller  Controller=PI  Form=Parallel  TimeDomain=Discrete-time  UseExternalTs=off  SampleTime=-1  IntegratorMethod=Forward Euler  FilterMethod=Forward Euler  ControllerParametersSource=external  P=single(350*40);  I=single(1200.0000*1/8e3)  UseKiTs=on  D=0  UseExternalDerivativeSource=off  N=100  UseFilter=off  TunerSelectOption=Transfer Function Based (PID Tuner App)  InitialConditionSource=external  InitialConditionForIntegrator=0  InitialConditionForFilter=0  DifferentiatorICPrevScaledInput=0  ExternalReset=level  TrackingMode=off  Kt=1  LimitOutput=on  SatLimitsSource=internal  UpperSaturationLimit=1e3  LowerSaturationLimit=-1e3  LinearizeAsGain=off  AntiWindupMode=none  Kb=1  LimitIntegrator=off  UpperIntegratorSaturationLimit=inf  LowerIntegratorSaturationLimit=-inf  POutMin=[]  POutMax=[]  IOutMin=[]  IOutMax=[]  DOutMin=[]  DOutMax=[]  NOutMin=[]  NOutMax=[]  SumOutMin=[]  SumOutMax=[]  SaturationOutMin=[]  SaturationOutMax=[]  PParamMin=[]  PParamMax=[]  IParamMin=[]  IParamMax=[]  DParamMin=[]  DParamMax=[]  NParamMin=[]  NParamMax=[]  KbParamMin=[]  KbParamMax=[]  KtParamMin=[]  KtParamMax=[]  KbOutMin=[]  KbOutMax=[]  KtOutMin=[]  KtOutMax=[]  IntegratorOutMin=[]  IntegratorOutMax=[]  FilterOutMin=[]  FilterOutMax=[]  SumI1OutMin=[]  SumI1OutMax=[]  SumI2OutMin=[]  SumI2OutMax=[]  SumI3OutMin=[]  SumI3OutMax=[]  SumI4OutMin=[]  SumI4OutMax=[]  SumDOutMin=[]  SumDOutMax=[]  DifferentiatorOutMin=[]  DifferentiatorOutMax=[]  FilterDiffOutCoefMin=[]  FilterDiffOutCoefMax=[]  ReciprocalOutMin=[]  ReciprocalOutMax=[]  SumDenOutMin=[]  SumDenOutMax=[]  SumNumOutMin=[]  SumNumOutMax=[]  DivideOutMin=[]  DivideOutMax=[]  UdiffTsProdOutMin=[]  UdiffTsProdOutMax=[]  NTsProdOutMin=[]  NTsProdOutMax=[]  UintegralTsProdOutMin=[]  UintegralTsProdOutMax=[]  UngainTsProdOutMin=[]  UngainTsProdOutMax=[]  ClampingZeroOutDataTypeStr=Inherit: Inherit via back propagation  ClampingZeroOutMin=[]  ClampingZeroOutMax=[]  FilterDenConstantOutDataTypeStr=Inherit: Inherit via back propagation  FilterDenConstantOutMin=[]  FilterDenConstantOutMax=[]  PCopyOutDataTypeStr=Inherit: Inherit via back propagation  PCopyOutMin=[]  PCopyOutMax=[]  NCopyOutDataTypeStr=Inherit: Inherit via back propagation  NCopyOutMin=[]  NCopyOutMax=[]  IntegratorContinuousStateAttributes=''  IntegratorStateMustResolveToSignalObject=off  IntegratorRTWStateStorageClass=Auto  FilterContinuousStateAttributes=''  FilterStateMustResolveToSignalObject=off  FilterRTWStateStorageClass=Auto  ParallelPVariant=ExternalParameters  IdealPVariant=Disabled  IVariant=ExternalParameters  DVariant=Disabled  IntegratorVariant=Discrete  SatVariant=Enabled  AWVariant=Passthrough  PCopyVariant=Disabled  TRVariant=Disabled  FdbkBlocksVariant=Forward  IdealPFdbkVariant=Disabled  SatFdbkVariant=Disabled  DerivativeFilterVariant=Disabled  NVariant=Disabled  NCopyVariant=Disabled_SignalSpec  FilterICVariant=Disabled  IntegratorICVariant=ExternalICs  ExternalResetVariant=ExternalReset  TRSumVariant=Passthrough  SumFdbkVariant=Disabled  SumVariant=Sum_PI  TsampFilterVariant=InternalTs  TsampNgainVariant=Passthrough  TsampIntegralVariant=Disabled_SignalSpec  ExternalSaturationOutDataTypeStr=Inherit: Same as second input  DerivativeSourceVariant=Disabled  PreIntVariant=InternalPreInt
      settings: LibrarySourceBlock=simulink/Discrete/Discrete PID Controller
  Gain : Gain  Commented=on  Gain=40  OutDataTypeStr=single
  Gain1 : Gain  Gain=(220*sqrt(2))
  Gain2 : Gain  Gain=(220*sqrt(2))
  Gain3 : Gain  Gain=3e2
  Gain4 : Gain  Gain=1/gain_vac  OutDataTypeStr=single
  Gain5 : Gain  Gain=1/gain_vac  OutDataTypeStr=single
  Memory1 : Memory  Commented=on  InheritSampleTime=on
  Memory2 : Memory  InitialCondition=.99  InheritSampleTime=on
  Memory3 : Memory  InheritSampleTime=on
  Memory4 : Memory  InheritSampleTime=on
  Park Transform : mcbcontrolslib/Park Transform  Commented=on  PhaseInput=Two inputs  AxisAlignment=Q-axis  ThetaInput=Sine and Cosine electrical position  AngleInput=Per-unit  N_points=1024
      settings: LibrarySourceBlock=mcbhdllib/Controls/Math Transforms/Park Transform
  Terminator{,1,3..4} (4 alike) : Terminator
  dco : MATLAB Function  TreatAsAtomicUnit=on  VariantControl=false()
  park_tf : MATLAB Function  TreatAsAtomicUnit=on  VariantControl=false()
  pi_ctrl : MATLAB Function  Commented=on  TreatAsAtomicUnit=on  VariantControl=false()
  vq_park_k_1 : Memory  Commented=on  InheritSampleTime=on
  angle : Outport
  vq_park : Outport  Port=2
  vd_park : Outport  Port=3
  sine : Outport  Port=4
  cos : Outport  Port=5
  w_lpf : Outport  Port=6
  vp_betha : Outport  Port=7
  vp_alpha : Outport  Port=8
  wires:
  Memory2/1 -> dco/1(cos_th_1)
  Memory1/1 -> pi_ctrl/3(w_pi_k_1)
  dco/1(th) -> Bias/1, Memory4/1  "angle"
  Beta/1 -> Park Transform/2, park_tf/2(vp_betha)
  Alpha/1 -> Park Transform/1, park_tf/1(vp_alpha)
  dco/3(cos_th) -> cos/1, Delay/1, Memory2/1  "cos_th"
  park_tf/2(vq_park) -> Gain5/1, Gain2/1, vq_park/1, vq_park_k_1/1, Gain3/1, pi_ctrl/1(vq_park)  "error_dsogi"
  vq_park_k_1/1 -> pi_ctrl/2(vq_park_k_1)
  dco/2(sin_th) -> sine/1, Delay1/1, Memory3/1  "sin_dco"
  park_tf/1(vd_park) -> Gain4/1, Gain1/1, vd_park/1  "vpark_d"
  Delay1/1 -> Park Transform/3, park_tf/3(sin_th_k_1)
  Memory4/1 -> dco/3(th_1)
  pi_ctrl/1(w_pi) -> Memory1/1, Gain/1
  Memory3/1 -> dco/2(sin_th_1)  "sin_th_1"
  Delay/1 -> Park Transform/4, park_tf/4(cos_th_k_1)
  Bias/1 -> angle/1
  Constant/1 -> ?  "w_fdbk"
  2nd_lp_filter/1(y) -> w_lpf/1  "w_"
  Gain1/1 -> Terminator/1  "vd_park_pll"
  Gain2/1 -> Terminator1/1  "vq_park_pll"
  Discrete PID Controller/1 -> dco/4(wo), 2nd_lp_filter/1(u)  "w_pid"
  Park Transform/2 -> Terminator3/1  "q_pll"
  Park Transform/1 -> Terminator4/1  "d_pll"
  Constant2/1 -> Discrete PID Controller/2  "w_fdbk"
  Gain3/1 -> Discrete PID Controller/1
  Constant1/1 -> Discrete PID Controller/4, Discrete PID Controller/5  "w_fdbk"
  Constant3/1 -> Discrete PID Controller/3  "w_fdbk"
  Gain4/1 -> vp_alpha/1
  Gain5/1 -> vp_betha/1

== system ctrl_ez/ctrl_ez_fcn/ctrl/pi_ctrl/id_ctrl ==
  i_error : Inport  OutDataTypeStr=single
  Accumulator : DiscreteIntegrator  IntegratorMethod=Accumulation: Backward Euler  gainval=1  SampleTime=-1  LimitOutput=on  UpperSaturationLimit=100  LowerSaturationLimit=-100  ShowSaturationPort=on  ICPrevOutput=DiscIntNeverNeededParam  ICPrevScaledInput=DiscIntNeverNeededParam
  Add2 : Sum
  Constant : Constant  Value=0  OutDataTypeStr=single  SampleTime=-1
  Delay : Delay
  Gain1 : Gain  Gain=kpd  OutDataTypeStr=single
  Gain2 : Gain  Gain=kid*tsw  OutDataTypeStr=single
  Saturation : Saturate  Commented=through  UpperLimit=350  LowerLimit=-500
  Switch : Switch  Criteria=u2 > Threshold  SaturateOnIntegerOverflow=off  InputSameDT=off
  v_ind : Outport
  wires:
  Gain1/1 -> Add2/1
  i_error/1 -> Gain2/1, Gain1/1  "int_id_fed"
  Accumulator/1 -> Add2/2  "id_integ"
  Gain2/1 -> Switch/3
  Switch/1 -> Accumulator/1
  Saturation/1 -> v_ind/1  "V_D_ind_ctrl"
  Delay/1 -> Switch/2
  Constant/1 -> Switch/1
  Add2/1 -> Saturation/1
  Accumulator/2 -> Delay/1

== system ctrl_ez/ctrl_ez_fcn/ctrl/pi_ctrl/iq_ctrl ==
  i_error : Inport  OutDataTypeStr=single
  Accumulator : DiscreteIntegrator  IntegratorMethod=Accumulation: Backward Euler  ExternalReset=rising  SampleTime=-1  LimitOutput=on  UpperSaturationLimit=500  LowerSaturationLimit=-500  ShowSaturationPort=on  ICPrevOutput=DiscIntNeverNeededParam  ICPrevScaledInput=DiscIntNeverNeededParam
  Add2 : Sum
  Constant1 : Constant  Value=0  OutDataTypeStr=single  SampleTime=-1
  Delay1 : Delay  DelayLength=1  InputProcessing=Columns as channels (frame based)
  Gain1 : Gain  Gain=kpq  OutDataTypeStr=single
  Gain2 : Gain  Gain=kiq*tsw  OutDataTypeStr=single
  Saturation : Saturate  Commented=through  UpperLimit=5  LowerLimit=-5
  Switch : Switch  Criteria=u2 > Threshold  SaturateOnIntegerOverflow=off  InputSameDT=off
  v_ind : Outport
  wires:
  i_error/1 -> Gain1/1, Switch/3  "error"
  Accumulator/2 -> Delay1/1
  Accumulator/1 -> Add2/2  "iq_integ"
  Constant1/1 -> Switch/1
  Switch/1 -> Gain2/1
  Delay1/1 -> Accumulator/2, Switch/2
  Gain1/1 -> Add2/1
  Gain2/1 -> Accumulator/1
  Add2/1 -> Saturation/1
  Saturation/1 -> v_ind/1  "V_Q_ind_ctrl"

== system ctrl_ez/ctrl_ez_fcn/ctrl/pi_ctrl/speed_ctrl ==
  i_error : Inport  OutDataTypeStr=single
  Accumulator : DiscreteIntegrator  IntegratorMethod=Accumulation: Forward Euler  SampleTime=-1  LimitOutput=on  UpperSaturationLimit=50  LowerSaturationLimit=-50  ShowSaturationPort=on  ICPrevOutput=DiscIntNeverNeededParam  ICPrevScaledInput=DiscIntNeverNeededParam
  Add2 : Sum
  Constant1 : Constant  Value=0  OutDataTypeStr=single  SampleTime=-1
  Delay1 : Delay  DelayLength=1  InputProcessing=Columns as channels (frame based)
  Gain1 : Gain  Gain=kpvdc  OutDataTypeStr=single
  Gain2 : Gain  Gain=kivdc  OutDataTypeStr=single
  Saturation : Saturate  UpperLimit=50  LowerLimit=-50
  Switch : Switch  Criteria=u2 > Threshold  SaturateOnIntegerOverflow=off  InputSameDT=off
  I_D_CTRL_VDC : Outport
  wires:
  i_error/1 -> Gain1/1, Switch/3  "error"
  Accumulator/2 -> Delay1/1
  Accumulator/1 -> Add2/2
  Constant1/1 -> Switch/1
  Switch/1 -> Gain2/1
  Delay1/1 -> Switch/2
  Gain1/1 -> Add2/1
  Gain2/1 -> Accumulator/1
  Add2/1 -> Saturation/1
  Saturation/1 -> I_D_CTRL_VDC/1  "I_D_CTRL_VDC"

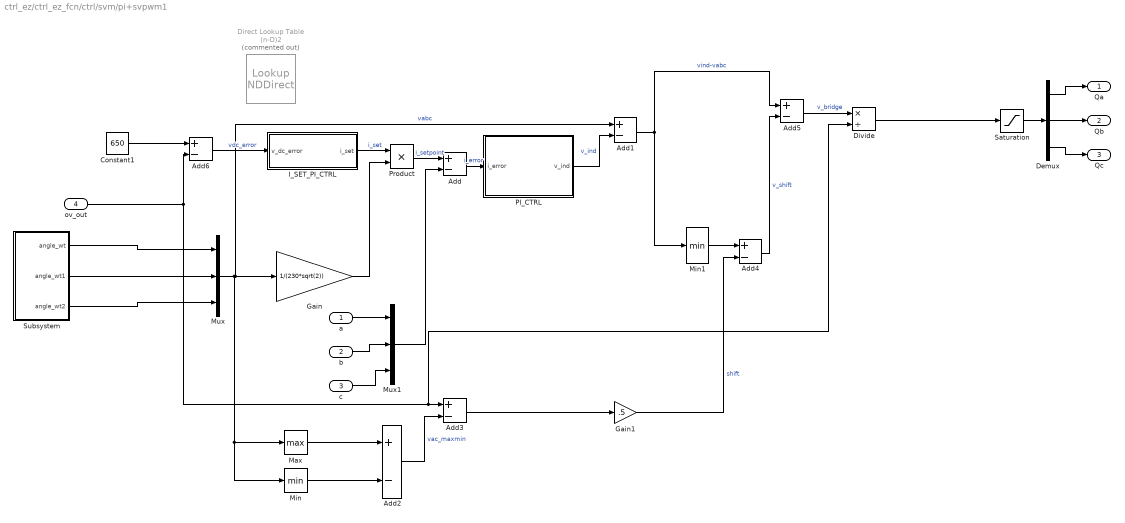
== system ctrl_ez/ctrl_ez_fcn/ctrl/svm/pi+svpwm1 ==
  a : Inport
  b : Inport  Port=2
  c : Inport  Port=3
  ov_out : Inport  Port=4
  Add{,1..6} (7 alike) : Sum  Inputs=+-
  Constant1 : Constant  Value=650  VectorParams1D=off  OutDataTypeStr=single  SampleTime=-1
  Demux : Demux  Outputs=3
  Direct Lookup Table (n-D)2 : LookupNDDirect  Commented=on  NumberOfTableDimensions=1  Table=single(cos_th);  RemoveProtectionInput=on  TableDataTypeStr=single
  Divide : Product  Inputs=*/
  Gain : Gain  Gain=1/(230*sqrt(2))
  Gain1 : Gain  Gain=.5
  I_SET_PI_CTRL : Subsystem  SystemSampleTime=tsw
  Max : MinMax  Function=max
  Min : MinMax
  Min1 : MinMax
  Mux : Mux  Inputs=3
  Mux1 : Mux  Inputs=3
  PI_CTRL : Subsystem  SystemSampleTime=tsw
  Product : Product
  Saturation : Saturate  UpperLimit=.97  LowerLimit=.03
  Subsystem : Subsystem
  Qa : Outport
  Qb : Outport  Port=2
  Qc : Outport  Port=3
  wires:
  Constant1/1 -> Add6/1
  ov_out/1 -> Add6/2, Divide/2, Add3/1
  Gain/1 -> Product/2
  Add6/1 -> I_SET_PI_CTRL/1(v_dc_error)  "vdc_error"
  b/1 -> Mux1/2
  Mux/1 -> Max/1, Min/1, Add1/1, Gain/1  "vabc"
  a/1 -> Mux1/1
  c/1 -> Mux1/3
  Max/1 -> Add2/1
  Min/1 -> Add2/2
  Product/1 -> Add/1  "i_setpoint"
  Mux1/1 -> Add/2
  Add2/1 -> Add3/2  "vac_maxmin"
  Add/1 -> PI_CTRL/1(i_error)  "i_error"
  Add3/1 -> Gain1/1
  PI_CTRL/1(v_ind) -> Add1/2  "v_ind"
  Add1/1 -> Add5/1, Min1/1  "vind-vabc"
  Gain1/1 -> Add4/2  "shift"
  Min1/1 -> Add4/1
  Add4/1 -> Add5/2  "v_shift"
  Add5/1 -> Divide/1  "v_bridge"
  Divide/1 -> Saturation/1
  Demux/2 -> Qb/1
  Demux/1 -> Qa/1
  Saturation/1 -> Demux/1
  Demux/3 -> Qc/1
  I_SET_PI_CTRL/1(i_set) -> Product/1  "i_set"
  Subsystem/1(angle_wt) -> Mux/1
  Subsystem/2(angle_wt1) -> Mux/2
  Subsystem/3(angle_wt2) -> Mux/3

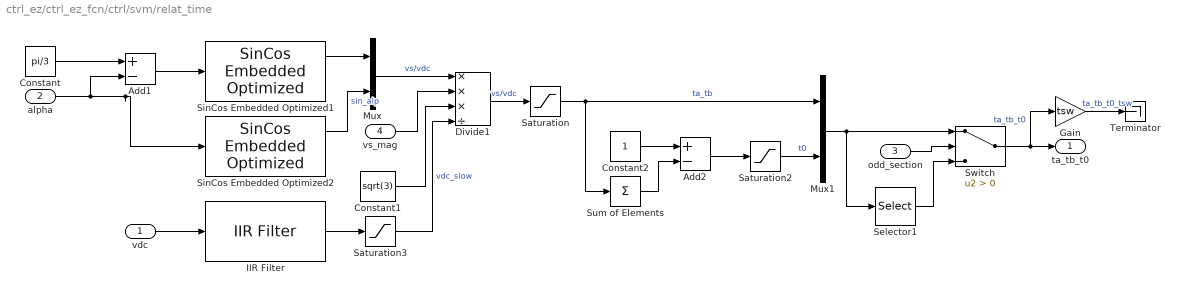
== system ctrl_ez/ctrl_ez_fcn/ctrl/svm/relat_time ==
  vdc : Inport
  alpha : Inport  Port=2
  odd_section : Inport  Port=3
  vs_mag : Inport  Port=4
  Add1 : Sum  Inputs=+-
  Add2 : Sum  Inputs=+-
  Constant : Constant  Value=pi/3  VectorParams1D=off  OutDataTypeStr=single  SampleTime=-1
  Constant1 : Constant  Value=sqrt(3)  VectorParams1D=off  OutDataTypeStr=single  SampleTime=-1
  Constant2 : Constant  VectorParams1D=off  OutDataTypeStr=single  SampleTime=-1
  Divide1 : Product  Inputs=***/
  Gain : Gain  Gain=tsw
  IIR Filter : mcbcontrolslib/IIR Filter  VariantControl=Low Pass Filter  VariantSelect=Low-pass  FilterConstantInputType=Specify via dialog  Filter_constant=0.01  advancedSettings=on  Ts=2*tsw  cutOff_freq=1
      settings: LibrarySourceBlock=mcbhdllib/Signal Management/IIR Filter
  Mux : Mux  Inputs=2
  Mux1 : Mux  Inputs=2
  Saturation : Saturate  UpperLimit=1  LowerLimit=0
  Saturation2 : Saturate  UpperLimit=1  LowerLimit=0
  Saturation3 : Saturate  UpperLimit=2000  LowerLimit=100
  Selector1 : Selector  InputPortWidth=3  IndexOptions=Index vector (dialog)  Indices=[2 1 3]  OutputSizes=1
  SinCos Embedded Optimized1 : mcbcontrolslib/SinCos Embedded Optimized  LabelModeActiveChoice=Sim_Sin  OptforProc=off  ApproximationMethod=None  UserApproxMethod=CORDIC  ApproxStatus=None  InterpMethod=Linear point-slope  NumberOfDataPoints=16  NumberOfIterations=11  RemoveProtectionAgainstOutOfRangeInput=off  TableDataTypeStr=Inherit: Inherit via input  AngleInput=Per-unit  ThetaDataType=single  N_points=1024  DatatypeInput=Inherit from input  Datatype=Inherit: Same as input
      settings: LibrarySourceBlock=mcblib/Controls/Math Transforms/SinCos Embedded Optimized
  SinCos Embedded Optimized2 : mcbcontrolslib/SinCos Embedded Optimized  LabelModeActiveChoice=Sim_Sin  OptforProc=off  ApproximationMethod=None  UserApproxMethod=CORDIC  ApproxStatus=None  InterpMethod=Linear point-slope  NumberOfDataPoints=16  NumberOfIterations=11  RemoveProtectionAgainstOutOfRangeInput=off  TableDataTypeStr=Inherit: Inherit via input  AngleInput=Per-unit  ThetaDataType=single  N_points=1024  DatatypeInput=Inherit from input  Datatype=Inherit: Same as input
      settings: LibrarySourceBlock=mcblib/Controls/Math Transforms/SinCos Embedded Optimized
  Sum of Elements : Sum  Inputs=+
  Switch : Switch  Criteria=u2 > Threshold  SaturateOnIntegerOverflow=off  InputSameDT=off
  Terminator : Terminator
  ta_tb_t0 : Outport
  wires:
  Constant1/1 -> Divide1/3
  vdc/1 -> IIR Filter/1
  Mux/1 -> Divide1/1  "vs/vdc"
  Sum of Elements/1 -> Add2/2
  Constant2/1 -> Add2/1
  alpha/1 -> SinCos Embedded Optimized2/1, Add1/2
  Add1/1 -> SinCos Embedded Optimized1/1
  Add2/1 -> Saturation2/1
  vs_mag/1 -> Divide1/2
  Constant/1 -> Add1/1
  SinCos Embedded Optimized1/1 -> Mux/1
  SinCos Embedded Optimized2/1 -> Mux/2  "sin_alp"
  IIR Filter/1 -> Saturation3/1
  Saturation3/1 -> Divide1/4  "vdc_slow"
  Divide1/1 -> Saturation/1  "vs/vdc"
  Saturation/1 -> Mux1/1, Sum of Elements/1  "ta_tb"
  odd_section/1 -> Switch/2
  Saturation2/1 -> Mux1/2  "t0"
  Mux1/1 -> Switch/1, Selector1/1
  Selector1/1 -> Switch/3
  Switch/1 -> Gain/1, ta_tb_t0/1  "ta_tb_t0"
  Gain/1 -> Terminator/1  "ta_tb_t0_tsw"

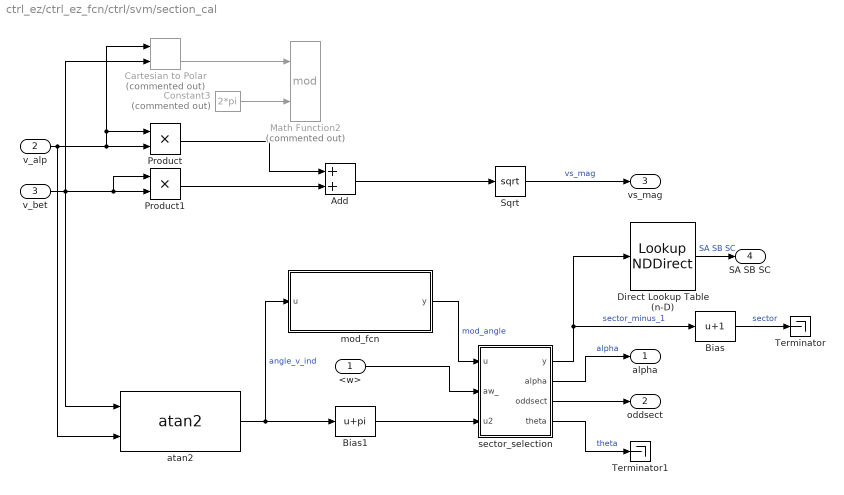
== system ctrl_ez/ctrl_ez_fcn/ctrl/svm/section_cal ==
  <w> : Inport
  v_alp : Inport  Port=2
  v_bet : Inport  Port=3
  Add : Sum
  Bias : Bias  Bias=1  SaturateOnIntegerOverflow=off
  Bias1 : Bias  Bias=pi  SaturateOnIntegerOverflow=off
  Cartesian to Polar : simulink_extras/Transformations/Cartesian to Polar  Commented=on
  Constant3 : Constant  Commented=on  Value=2*pi  OutDataTypeStr=single  SampleTime=-1
  Direct Lookup Table (n-D) : LookupNDDirect  InputsSelectThisObjectFromTable=Vector  Table=[3 2 1 1 2 3;2 3 3 2 1 1;1 1 2 3 3 2]  RemoveProtectionInput=on  TableDataTypeStr=single
  Math Function2 : Math  Commented=on  Operator=mod  SignedPower=on  OutputSignalType=real
  Product : Product
  Product1 : Product
  Sqrt : Sqrt  OutputSignalType=real
  Terminator : Terminator
  Terminator1 : Terminator
  atan2 : mcbcontrolslib/atan2  ApproximationMethod=Lookup  NumberOfIterations=11  NumberOfDataPoints=16  InterpMethod=Linear point-slope  outputUnit=Radians  TableDataTypeStr=single
      settings: LibrarySourceBlock=mcblib/Controls/Math Transforms/atan2
  mod_fcn : MATLAB Function  TreatAsAtomicUnit=on
  sector_selection : MATLAB Function  TreatAsAtomicUnit=on
  alpha : Outport
  oddsect : Outport  Port=2
  vs_mag : Outport  Port=3
  SA SB SC : Outport  Port=4
  wires:
  Product/1 -> Add/1
  <w>/1 -> sector_selection/2(aw_)
  v_alp/1 -> Product/1, Cartesian to Polar/1, Product/2, atan2/2
  Product1/1 -> Add/2
  v_bet/1 -> Product1/1, Product1/2, atan2/1, Cartesian to Polar/2
  Cartesian to Polar/2 -> Math Function2/1
  Constant3/1 -> Math Function2/2
  mod_fcn/1(y) -> sector_selection/1(u)  "mod_angle"
  atan2/1 -> Bias1/1, mod_fcn/1(u)  "angle_v_ind"
  Add/1 -> Sqrt/1
  Bias/1 -> Terminator/1  "sector"
  Bias1/1 -> sector_selection/3(u2)
  Sqrt/1 -> vs_mag/1  "vs_mag"
  sector_selection/3(oddsect) -> oddsect/1
  sector_selection/2(alpha) -> alpha/1  "alpha"
  sector_selection/1(y) -> Direct Lookup Table (n-D)/1, Bias/1  "sector_minus_1"
  sector_selection/4(theta) -> Terminator1/1  "theta"
  Direct Lookup Table (n-D)/1 -> SA SB SC/1  "SA SB SC"

== system ctrl_ez/ctrl_ez_fcn/ctrl/svm/threshold ==
  ta_tb_t0 : Inport
  SA SB SC : Inport  Port=2
  Add3 : Sum
  Add4 : Sum
  Demux : Demux  Outputs=3
  Demux1 : Demux  Outputs=3
  Gain : Gain  Gain=.5
  Mux : Mux  Inputs=3
      settings: DisplayOption=signals
  Saturation1 : Saturate  UpperLimit=.97  LowerLimit=.03
  Saturation4 : Saturate  UpperLimit=1  LowerLimit=0
  Saturation5 : Saturate  UpperLimit=1  LowerLimit=0
  Selector : Selector  InputPortWidth=3  IndexOptions=Index vector (port)  Indices=[1 3]  OutputSizes=1
  qa : Outport
  qb : Outport  Port=2
  qc : Outport  Port=3
  wires:
  Demux1/3 -> Gain/1
  ta_tb_t0/1 -> Demux1/1
  Add4/1 -> Saturation5/1  "T3"
  SA SB SC/1 -> Selector/2
  Saturation4/1 -> Add4/2, Mux/2  "T2"
  Add3/1 -> Saturation4/1  "T2"
  Demux1/1 -> Add4/1
  Gain/1 -> Mux/1, Add3/2  "T1"
  Demux1/2 -> Add3/1
  Saturation5/1 -> Mux/3  "T3"
  Mux/1 -> Selector/1
  Selector/1 -> Saturation1/1
  Saturation1/1 -> Demux/1  "T2"
  Demux/1 -> qa/1
  Demux/2 -> qb/1
  Demux/3 -> qc/1
